simulink model "testV2"  (R2018a)
settings: Solver=VariableStepAuto  StartTime=0.0  StopTime=inf  RelTol=1e-3  EnableMultiTasking=on
libraries: aerolibanimutils x1
settings Model: Creator=santd  LastModifiedBy=robotnuc
settings OptimizationCC: LifeSpan=inf
settings DebuggingCC: SFUnexpectedBacktrackingDiag=warning  SFNoUnconditionalDefaultTransitionDiag=warning  SFExecutionAtInitializationDiag=none
settings CodeAppCC: StateflowObjectComments=on
settings GRTTargetCC: TargetLangStandard=C89/C90 (ANSI)  GeneratePreprocessorConditionals=Disable all
settings ConfigComp: CovMetricSettings=dw  CovHtmlReporting=on  CovSaveCumulativeToWorkspaceVar=on  CovSaveSingleToWorkspaceVar=on  CovExternalEMLEnable=off

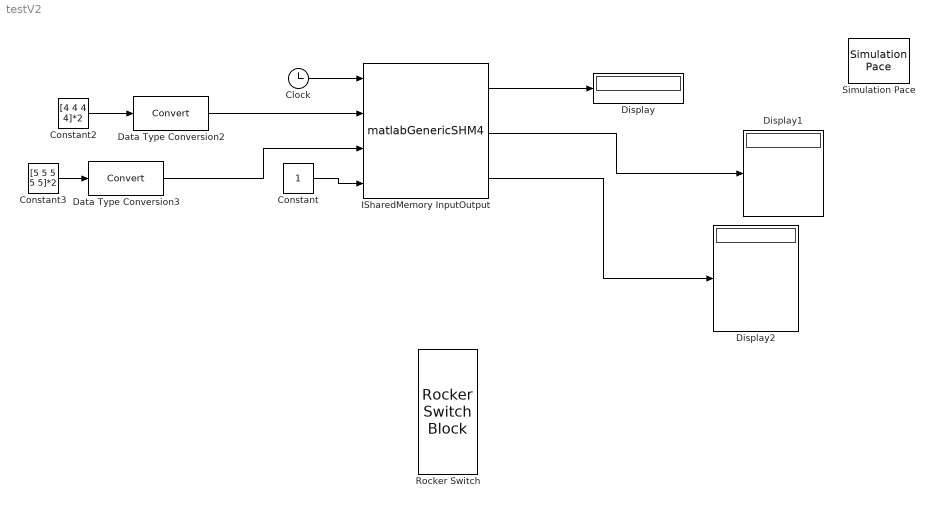
== system testV2 ==
  Clock : Clock
  Constant : Constant
  Constant2 : Constant  Value=[4 4 4 4]*2
  Constant3 : Constant  Value=[5 5 5 5 5]*2
  Data Type Conversion2 : DataTypeConversion
  Data Type Conversion3 : DataTypeConversion
  Display : Display
  Display1 : Display
  Display2 : Display
  ISharedMemory InputOutput : S-Function  FunctionName=matlabGenericSHM4  Parameters=nameIn,nameOut,vecE,vecS,tipoE,tipoS,ts,trigg,inOff,outOff  SFunctionDeploymentMode=off  EnableBusSupport=off  mask(ISharedMemory InputOutput (Generic Share Memory block V3.0)){nameIn='input_in', nameOut='input_in', vecE=[1 4 5], vecS=[1 4 5], tipoE=['d' 'd' 'd'], tipoS=['d' 'd' 'd'], inOff=0, outOff=0, ts=-1, trigg=on}
      mask prompts: nameIn "Input Shared Memory Name"; nameOut "Output Shared Memory Name"; vecE "Vector of system inputs"; vecS "Vector of system outputs"; tipoE "Data Types Inputs"; tipoS "Data Types Outputs"; inOff "Input Shared Memory Offset"; outOff "Output Shared Memory Offset"; ts "Sample Time"; trigg "Triggered writing"
      mask help:
      | This block allows Simulink communication with external processes through shared memory. It works on Unix and Windows.
      | More information in Help.
      mask Help:
      | Input Shared Memory Name: Name of the memory from which the physical device acquires its inputs.
      | Output Shared Memory Name: Name of the memory in which the physical device writes its output data.
      | Vector of system inputs: array that specify the number of inputs (array dimension) and the inputs size (array values)
      | Vector of system outputs: array that specify the number of outputs (array dimension) and the outputs size (array values)
      | Data types input: char array that specify each input types
      | Data types output: char array that specify each output types
      | Allowed types are:
      | ('f'=float, 'd'=double, 'i'=int32, 'c'=char, 'C'= unsigned char, 'I'=unsigned int)
      | 
      | Imput Shared Memory Offset: Position (in bytes) from which data is written into the input memory to the device.
      | Output Shared Memory Offset: Position (in bytes) from which the data from the output memory of the device is read.
      | Note: the final size of the memory is equal to the amount of I/O multiplied by the size of each I/O plus the offset. For example, a memory with size=[2 3] , type =['f' 'c'] and offset = 10 will have a final size of 2 * 4 + 3 * 1 + 10 = 21 bytes, although only the 2*4 +3*1 = 11 last bytes are used.
      | 
      | Triggered writing: If trigger writing is selected, an additional block input is created at the end of inputs. When this input has a value greater than zero the data at the input of the block is written to the device input shared memory, otherwise the data is not written.
      | 
      | Sample Time: Explicit block sampling time.
      | 
      | Example.
      | Suppose the following parameters:
      | Input Shared Memory Name = "devIn_1"
      | Output Shared Memory Name = "devOut_1"
      | Vector of system inputs=[3 2 1]
      | Vector of system outputs=[6 5 7 8]
      | Data types output=['f' 'I' 'c']
      | tipoS=['C' 'i' 'd' 'd']
      | Imput Shared Memory Offset = 10
      | Output Shared Memory Offset =0
      | 
      | Two Share Memories are created with names:
      | "devIn_1"(block input)
      | "devOut_1"  (block output)
      | 3 inputs are created:
      |  1° Dimension 3, type "unsigned char"
      |  2° Dimension 2, type "int"
      |  3° Dimension 1, type "char"
      | 4 outputs are created:
      |  1° Dimension 6, type "float"
      |  2° Dimension 5, type "unsigned int"
      |  3° Dimension 7, type "double"
      |  3° Dimension 8, type "double"
      mask Display: image('mem4.png')
  Rocker Switch : RockerSwitchBlock  WebBlockId=24
      settings: Values={{'Off', 'On'}, [0 1]}
  Simulation Pace : aerolibanimutils/Simulation Pace  SimulationPace=1  SleepMode=MATLAB Thread  OutputPaceError=off  SampleTime=1/30
  wires:
  ISharedMemory InputOutput/1 -> Display/1
  Constant2/1 -> Data Type Conversion2/1
  Data Type Conversion2/1 -> ISharedMemory InputOutput/2
  Constant3/1 -> Data Type Conversion3/1
  Data Type Conversion3/1 -> ISharedMemory InputOutput/3
  Clock/1 -> ISharedMemory InputOutput/1
  ISharedMemory InputOutput/2 -> Display1/1
  ISharedMemory InputOutput/3 -> Display2/1
  Constant/1 -> ISharedMemory InputOutput/4
